simulink model "AXI_QPSK_Tx"  (R2017b)
settings: Solver=FixedStepAuto  StartTime=0.0  StopTime=1000/Rb  RelTol=1e-3
PreLoadFcn:
  | Rb = 10000;   % 1kbit / s
  | Rsym = Rb/2;   % 2 bits per symbol
  | Rsymbol = Rb/2;
  | OSR = 32;
  | f_error = 120;
  | 
  | design_filters_tx
values from neighbouring files (symbols this model uses):
  CIC_fine_Tx = 2^-(CIC_right_shift - CIC_left_shift - CIC_shift_Tx)    [design_filters_tx.m]
  fCIC = fCICcomp * R_CIC    (= 25600000)    [design_filters_tx.m]
  fHB = fRRC * R_HB    (= 40000)    [design_filters_tx.m]
  R_CIC = 320    [design_filters_tx.m]
  R_CICcomp = 2    [design_filters_tx.m]
  R_HB = 2    [design_filters_tx.m]
  R_RRC = 4    [design_filters_tx.m]
undefined symbols (not defined in the file or in its folder): AXI4, Lite
libraries: xbsIndex_r4 x281, hdlsllib x2
(part 2 of 3)

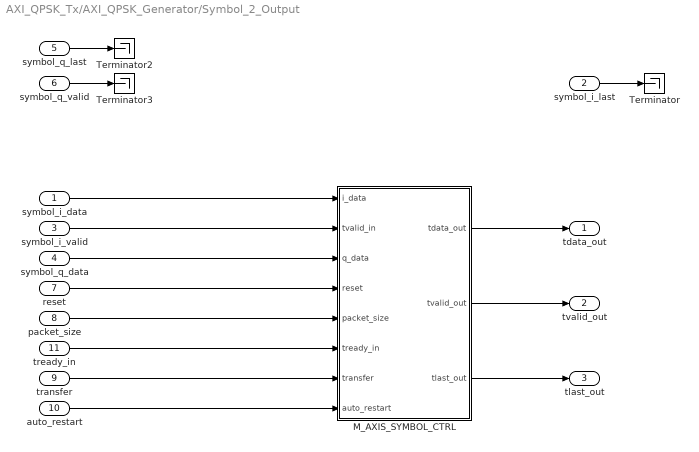
== system AXI_QPSK_Tx/AXI_QPSK_Generator/Symbol_2_Output ==
  symbol_i_data : Inport
  symbol_i_last : Inport  Port=2
  symbol_i_valid : Inport  Port=3
  symbol_q_data : Inport  Port=4
  symbol_q_last : Inport  Port=5
  symbol_q_valid : Inport  Port=6
  reset : Inport  Port=7
  packet_size : Inport  Port=8
  transfer : Inport  Port=9
  auto_restart : Inport  Port=10
  tready_in : Inport  Port=11
  M_AXIS_SYMBOL_CTRL : Subsystem
  Terminator : Terminator
  Terminator2 : Terminator
  Terminator3 : Terminator
  tdata_out : Outport
  tvalid_out : Outport  Port=2
  tlast_out : Outport  Port=3
  wires:
  symbol_i_last/1 -> Terminator/1
  symbol_q_last/1 -> Terminator2/1
  symbol_q_valid/1 -> Terminator3/1
  symbol_i_data/1 -> M_AXIS_SYMBOL_CTRL/1(i_data)
  symbol_i_valid/1 -> M_AXIS_SYMBOL_CTRL/2(tvalid_in)
  symbol_q_data/1 -> M_AXIS_SYMBOL_CTRL/3(q_data)
  reset/1 -> M_AXIS_SYMBOL_CTRL/4(reset)
  packet_size/1 -> M_AXIS_SYMBOL_CTRL/5(packet_size)
  tready_in/1 -> M_AXIS_SYMBOL_CTRL/6(tready_in)
  M_AXIS_SYMBOL_CTRL/1(tdata_out) -> tdata_out/1
  M_AXIS_SYMBOL_CTRL/2(tvalid_out) -> tvalid_out/1
  M_AXIS_SYMBOL_CTRL/3(tlast_out) -> tlast_out/1
  transfer/1 -> M_AXIS_SYMBOL_CTRL/7(transfer)
  auto_restart/1 -> M_AXIS_SYMBOL_CTRL/8(auto_restart)

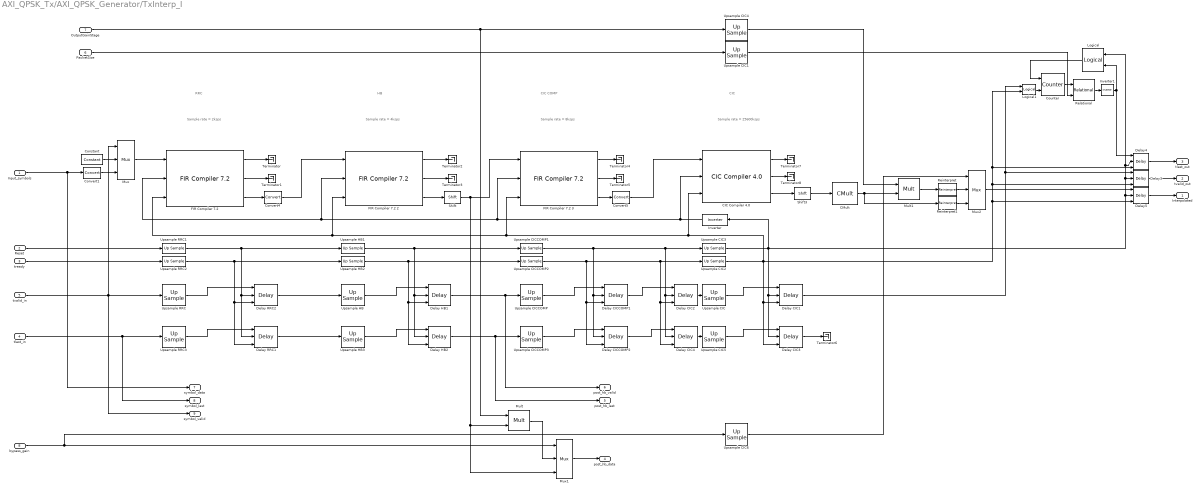
== system AXI_QPSK_Tx/AXI_QPSK_Generator/TxInterp_I ==
  note: HB
  note: RRC
  note: CIC COMP
  note: CIC
  note: Sample rate
      | = 2ksps
  note: Sample rate
      | = 4ksps
  note: Sample rate
      | = 8ksps
  note: Sample rate
      | = 25600ksps
  Input_symbols : Inport
  Reset : Inport  Port=2
  tready : Inport  Port=3
  tlast_in : Inport  Port=4
  tvalid_in : Inport  Port=5
  PacketSize : Inport  Port=6
  OutputGainStage : Inport  Port=7
  bypass_gain : Inport  Port=8
  "CIC Compiler 4.0 " : xbsIndex_r4/CIC Compiler 4.0   filter_type=Interpolation  number_of_stages=5  differential_delay=1  number_of_channels=1  sample_rate_changes=Fixed  fixed_or_initial_rate=R_CIC  minimum_rate=3200  maximum_rate=3200  ratespecification=Maximum_Possible  sampleperiod=3200  hardwareoversamplingrate=1  quantization=Full_Precision  output_data_width=65  use_xtreme_dsp_slice=on  use_streaming_interface=on  has_aclken=on  has_aresetn=on  has_dout_tready=off  trim_axipin_name=on  gui_behaviour=Sysgen_GUI  input_data_width=18  ip_name=CIC Compiler  ip_version=4.0  dsptool_ready=true  wrapper_available=true  port_translation_map={ 'aclken' => 'en', 'aresetn' => 'rst' }  ipcore_xco_need_fpga_part=true  ipcore_verbose=false  block_type=cic_compiler_v4_0
  CMult : xbsIndex_r4/CMult  const=CIC_fine_Tx  gui_display_data_type=Fixed-point  const_n_bits=16  const_bin_pt=15  float_type=Single  exp_bits=8  fraction_bits=24  en=off  latency=0  precision=User Defined  arith_type="Signed  (2's comp)"  n_bits=16  bin_pt=15  quantization=Truncate  overflow=Wrap  use_behavioral_HDL=off  mem_type=Distributed RAM  pipeline=off  dbl_ovrd=off  block_type=cmult
  Constant : xbsIndex_r4/Constant  const=0  gui_display_data_type=Fixed-point  arith_type=Signed (2's comp)  n_bits=16  bin_pt=0  preci_type=Single  exp_width=8  frac_width=24  explicit_period=on  period=2/Rb  equ=P=C  opselect=C  inp2=PCIN>>17  opr=+  inp1=P  carry=CIN  dbl_ovrd=off  block_type=constant
  Convert1 : xbsIndex_r4/Convert  gui_display_data_type=Fixed-point  arith_type="Signed  (2's comp)"  n_bits=16  bin_pt=0  float_type=Single  exp_bits=8  fraction_bits=24  quantization=Truncate  overflow=Wrap  en=off  latency=0  pipeline=off  dbl_ovrd=off  block_type=convert
  Convert4 : xbsIndex_r4/Convert  gui_display_data_type=Fixed-point  arith_type="Signed  (2's comp)"  n_bits=16  bin_pt=15  float_type=Single  exp_bits=8  fraction_bits=24  quantization=Truncate  overflow=Wrap  en=off  latency=0  pipeline=off  dbl_ovrd=off  block_type=convert
  Convert5 : xbsIndex_r4/Convert  gui_display_data_type=Fixed-point  arith_type="Signed  (2's comp)"  n_bits=16  bin_pt=15  float_type=Single  exp_bits=8  fraction_bits=24  quantization=Truncate  overflow=Wrap  en=off  latency=0  pipeline=off  dbl_ovrd=off  block_type=convert
  Counter : xbsIndex_r4/Counter  cnt_type=Free Running  cnt_to=Inf  operation=Up  start_count=0  cnt_by_val=1  arith_type=Unsigned  n_bits=32  bin_pt=0  load_pin=off  rst=on  en=on  explicit_period=on  period=1/fCIC  use_behavioral_HDL=off  implementation=Fabric  dbl_ovrd=off  block_type=counter
  Delay CIC1 : xbsIndex_r4/Delay  rst=on  infoeditControl=Selection of Reset will increase slice count due to use of real FFs and instead of SRLs  en=on  latency=3*8  reg_retiming=off  dbl_ovrd=off  block_type=delay
  Delay CIC2 : xbsIndex_r4/Delay  rst=on  infoeditControl=Selection of Reset will increase slice count due to use of real FFs and instead of SRLs  en=on  latency=4  reg_retiming=off  dbl_ovrd=off  block_type=delay
  Delay CIC3 : xbsIndex_r4/Delay  rst=on  infoeditControl=Selection of Reset will increase slice count due to use of real FFs and instead of SRLs  en=on  latency=3*8-1  reg_retiming=off  dbl_ovrd=off  block_type=delay
  Delay CIC4 : xbsIndex_r4/Delay  rst=on  infoeditControl=Selection of Reset will increase slice count due to use of real FFs and instead of SRLs  en=on  latency=5  reg_retiming=off  dbl_ovrd=off  block_type=delay
  Delay CICCOMP1 : xbsIndex_r4/Delay  rst=on  infoeditControl=Selection of Reset will increase slice count due to use of real FFs and instead of SRLs  en=on  latency=R_CICcomp*4  reg_retiming=off  dbl_ovrd=off  block_type=delay
  Delay CICCOMP2 : xbsIndex_r4/Delay  rst=on  infoeditControl=Selection of Reset will increase slice count due to use of real FFs and instead of SRLs  en=on  latency=R_CICcomp*4+1  reg_retiming=off  dbl_ovrd=off  block_type=delay
  Delay HB1 : xbsIndex_r4/Delay  rst=on  infoeditControl=Selection of Reset will increase slice count due to use of real FFs and instead of SRLs  en=on  latency=R_HB*2  reg_retiming=off  dbl_ovrd=off  block_type=delay
  Delay HB2 : xbsIndex_r4/Delay  rst=on  infoeditControl=Selection of Reset will increase slice count due to use of real FFs and instead of SRLs  en=on  latency=R_HB*2+1  reg_retiming=off  dbl_ovrd=off  block_type=delay
  Delay RRC1 : xbsIndex_r4/Delay  rst=on  infoeditControl=Selection of Reset will increase slice count due to use of real FFs and instead of SRLs  en=on  latency=3*R_RRC  reg_retiming=off  dbl_ovrd=off  block_type=delay
  Delay RRC2 : xbsIndex_r4/Delay  rst=on  infoeditControl=Selection of Reset will increase slice count due to use of real FFs and instead of SRLs  en=on  latency=R_RRC*2+1  reg_retiming=off  dbl_ovrd=off  block_type=delay
  Delay3 : xbsIndex_r4/Delay  rst=on  infoeditControl=Selection of Reset will increase slice count due to use of real FFs and instead of SRLs  en=on  latency=1  reg_retiming=off  dbl_ovrd=off  block_type=delay
  Delay4 : xbsIndex_r4/Delay  rst=on  infoeditControl=Selection of Reset will increase slice count due to use of real FFs and instead of SRLs  en=on  latency=1  reg_retiming=off  dbl_ovrd=off  block_type=delay
  Delay5 : xbsIndex_r4/Delay  rst=on  infoeditControl=Selection of Reset will increase slice count due to use of real FFs and instead of SRLs  en=on  latency=1  reg_retiming=off  dbl_ovrd=off  block_type=delay
  "FIR Compiler 7.2 " : xbsIndex_r4/FIR Compiler 7.2   coefficientvector=WRRC.Numerator  coefficient_sets=1  coefficient_reload=off  filter_type=Interpolation  rate_change_type=Integer  interpolation_rate=R_RRC  decimation_rate=1  zero_pack_factor=1  channel_sequence=Basic  number_channels=1  pattern_list='P4-0,P4-1,P4-2,P4-3,P4-4'  number_paths=1  ratespecification=Maximum_Possible  sampleperiod=1  hardwareoversamplingrate=1  coefficient_sign=Signed  quantization=Quantize_Only  coefficient_width=16  bestprecision=on  coefficient_fractional_bits=15  coefficient_structure=Inferred  output_rounding_mode=Full_Precision  output_width=31  filter_architecture=Systolic_Multiply_Accumulate  optimization_goal=Area  optimization_list='None'  data_buffer_type=Automatic  coefficient_buffer_type=Automatic  input_buffer_type=Automatic  output_buffer_type=Automatic  preference_for_other_storage=Automatic  multi_column_support=Automatic  columnconfig='13'  inter_column_pipe_length=4  data_has_tlast=Not_Required  m_data_has_tready=off  s_data_has_fifo=off  s_data_has_tuser=Not_Required  m_data_has_tuser=Not_Required  s_config_sync_mode=On_Vector  s_config_method=Single  num_reload_slots=1  has_aclken=on  has_aresetn=on  infoeditControl=ARESETn must be asserted for a minimum of 2 cycles  reset_data_vector=on  trim_axipin_name=on  simulation_type=hybrid_sim  simulation_model=sysgen:xfirv7_2_cmodel  data_path_portlist={ 's_axis_data_tdata', 'm_axis_data_tdata' }  passband_min=0.0  passband_max=0.5  stopband_min=0.5  stopband_max=1.0  filter_selection=1  gui_behaviour='Sysgen_GUI'  data_sign=Signed  data_width=16  data_fractional_bits=0  data_tuser_width=1  wrapper_available=true  ip_wrap_arbitrary_binary_point=true  ip_name=FIR Compiler  ip_version=7.2  dsptool_ready=true  ipcore_usecache=true  ipcore_useipmodelcache=true  port_translation_map={ 'aclken' => 'en', 'aresetn' => 'rst' }  run_core_at_system_period=true  ipcore_xco_need_fpga_part=true  block_type=fir_compiler_v7_2
      settings: infoedit=Maximum Possible : Maximizes oversampling rate. Abstracted input handshake (no s_data_tvalid) and automatic rate propagation.<br>Hardware Oversampling Rate : Specifies oversampling rate relative to the input sample period. Abstracted input handshake (no s_data_tvalid) and automatic rate propagation.<br>Input/Output Sample Period : Specifies absolute oversampling rate. No input handshake abstraction (exposes s_data_tvalid) and no rate propagation.
  FIR Compiler 7.2 2 : xbsIndex_r4/FIR Compiler 7.2   coefficientvector=HB.Numerator  coefficient_sets=1  coefficient_reload=off  filter_type=Interpolation  rate_change_type=Integer  interpolation_rate=2  decimation_rate=1  zero_pack_factor=1  channel_sequence=Basic  number_channels=1  pattern_list='P4-0,P4-1,P4-2,P4-3,P4-4'  number_paths=1  ratespecification=Maximum_Possible  sampleperiod=1  hardwareoversamplingrate=1  coefficient_sign=Signed  quantization=Quantize_Only  coefficient_width=16  bestprecision=on  coefficient_fractional_bits=15  coefficient_structure=Inferred  output_rounding_mode=Full_Precision  output_width=32  filter_architecture=Systolic_Multiply_Accumulate  optimization_goal=Area  optimization_list='None'  data_buffer_type=Automatic  coefficient_buffer_type=Automatic  input_buffer_type=Automatic  output_buffer_type=Automatic  preference_for_other_storage=Automatic  multi_column_support=Automatic  columnconfig='6'  inter_column_pipe_length=4  data_has_tlast=Not_Required  m_data_has_tready=off  s_data_has_fifo=off  s_data_has_tuser=Not_Required  m_data_has_tuser=Not_Required  s_config_sync_mode=On_Vector  s_config_method=Single  num_reload_slots=1  has_aclken=on  has_aresetn=on  infoeditControl=ARESETn must be asserted for a minimum of 2 cycles  reset_data_vector=on  trim_axipin_name=on  simulation_type=hybrid_sim  simulation_model=sysgen:xfirv7_2_cmodel  data_path_portlist={ 's_axis_data_tdata', 'm_axis_data_tdata' }  passband_min=0.0  passband_max=0.5  stopband_min=0.5  stopband_max=1.0  filter_selection=1  gui_behaviour='Sysgen_GUI'  data_sign=Signed  data_width=16  data_fractional_bits=0  data_tuser_width=1  wrapper_available=true  ip_wrap_arbitrary_binary_point=true  ip_name=FIR Compiler  ip_version=7.2  dsptool_ready=true  ipcore_usecache=true  ipcore_useipmodelcache=true  port_translation_map={ 'aclken' => 'en', 'aresetn' => 'rst' }  run_core_at_system_period=true  ipcore_xco_need_fpga_part=true  block_type=fir_compiler_v7_2
      settings: infoedit=Maximum Possible : Maximizes oversampling rate. Abstracted input handshake (no s_data_tvalid) and automatic rate propagation.<br>Hardware Oversampling Rate : Specifies oversampling rate relative to the input sample period. Abstracted input handshake (no s_data_tvalid) and automatic rate propagation.<br>Input/Output Sample Period : Specifies absolute oversampling rate. No input handshake abstraction (exposes s_data_tvalid) and no rate propagation.
  FIR Compiler 7.2 3 : xbsIndex_r4/FIR Compiler 7.2   coefficientvector=WComp.Numerator  coefficient_sets=1  coefficient_reload=off  filter_type=Interpolation  rate_change_type=Integer  interpolation_rate=R_CICcomp  decimation_rate=1  zero_pack_factor=1  channel_sequence=Basic  number_channels=1  pattern_list='P4-0,P4-1,P4-2,P4-3,P4-4'  number_paths=1  ratespecification=Maximum_Possible  sampleperiod=1  hardwareoversamplingrate=1  coefficient_sign=Signed  quantization=Quantize_Only  coefficient_width=16  bestprecision=on  coefficient_fractional_bits=15  coefficient_structure=Inferred  output_rounding_mode=Full_Precision  output_width=33  filter_architecture=Systolic_Multiply_Accumulate  optimization_goal=Area  optimization_list='None'  data_buffer_type=Automatic  coefficient_buffer_type=Automatic  input_buffer_type=Automatic  output_buffer_type=Automatic  preference_for_other_storage=Automatic  multi_column_support=Automatic  columnconfig='19'  inter_column_pipe_length=4  data_has_tlast=Not_Required  m_data_has_tready=off  s_data_has_fifo=off  s_data_has_tuser=Not_Required  m_data_has_tuser=Not_Required  s_config_sync_mode=On_Vector  s_config_method=Single  num_reload_slots=1  has_aclken=on  has_aresetn=on  infoeditControl=ARESETn must be asserted for a minimum of 2 cycles  reset_data_vector=on  trim_axipin_name=on  simulation_type=hybrid_sim  simulation_model=sysgen:xfirv7_2_cmodel  data_path_portlist={ 's_axis_data_tdata', 'm_axis_data_tdata' }  passband_min=0.0  passband_max=0.5  stopband_min=0.5  stopband_max=1.0  filter_selection=1  gui_behaviour='Sysgen_GUI'  data_sign=Signed  data_width=16  data_fractional_bits=0  data_tuser_width=1  wrapper_available=true  ip_wrap_arbitrary_binary_point=true  ip_name=FIR Compiler  ip_version=7.2  dsptool_ready=true  ipcore_usecache=true  ipcore_useipmodelcache=true  port_translation_map={ 'aclken' => 'en', 'aresetn' => 'rst' }  run_core_at_system_period=true  ipcore_xco_need_fpga_part=true  block_type=fir_compiler_v7_2
      settings: infoedit=Maximum Possible : Maximizes oversampling rate. Abstracted input handshake (no s_data_tvalid) and automatic rate propagation.<br>Hardware Oversampling Rate : Specifies oversampling rate relative to the input sample period. Abstracted input handshake (no s_data_tvalid) and automatic rate propagation.<br>Input/Output Sample Period : Specifies absolute oversampling rate. No input handshake abstraction (exposes s_data_tvalid) and no rate propagation.
  Inverter : xbsIndex_r4/Inverter  en=off  latency=0  dbl_ovrd=off  block_type=inv
  Inverter1 : xbsIndex_r4/Inverter  en=off  latency=0  dbl_ovrd=off  block_type=inv
  Logical : xbsIndex_r4/Logical  logical_function=OR  inputs=2  en=off  latency=0  precision=Full  arith_type=Unsigned  n_bits=16  bin_pt=0  align_bp=on  dbl_ovrd=off  block_type=logical
  Logical1 : xbsIndex_r4/Logical  logical_function=AND  inputs=2  en=off  latency=0  precision=Full  arith_type=Unsigned  n_bits=16  bin_pt=0  align_bp=on  dbl_ovrd=off  block_type=logical
  Mult : xbsIndex_r4/Mult  precision=User Defined  arith_type="Signed  (2's comp)"  n_bits=16  bin_pt=15  quantization=Truncate  overflow=Wrap  en=off  latency=0  use_behavioral_HDL=off  opt=Speed  use_embedded=on  optimum_pipeline=off  pipeline=on  dbl_ovrd=off  use_rpm=on  placement_style=Triangular  block_type=mult
  Mult1 : xbsIndex_r4/Mult  precision=User Defined  arith_type="Signed  (2's comp)"  n_bits=16  bin_pt=15  quantization=Truncate  overflow=Wrap  en=off  latency=0  use_behavioral_HDL=off  opt=Speed  use_embedded=on  optimum_pipeline=off  pipeline=on  dbl_ovrd=off  use_rpm=on  placement_style=Triangular  block_type=mult
  Mux : xbsIndex_r4/Mux  inputs=2  en=off  latency=0  precision=Full  arith_type=Unsigned  n_bits=16  bin_pt=14  quantization=Truncate  overflow=Wrap  dbl_ovrd=off  block_type=mux
  Mux1 : xbsIndex_r4/Mux  inputs=2  en=off  latency=0  precision=Full  arith_type=Unsigned  n_bits=16  bin_pt=14  quantization=Truncate  overflow=Wrap  dbl_ovrd=off  block_type=mux
  Mux2 : xbsIndex_r4/Mux  inputs=2  en=off  latency=0  precision=Full  arith_type=Unsigned  n_bits=16  bin_pt=14  quantization=Truncate  overflow=Wrap  dbl_ovrd=off  block_type=mux
  Reinterpret : xbsIndex_r4/Reinterpret  force_arith_type=on  arith_type=Unsigned  force_bin_pt=on  bin_pt=0  block_type=reinterpret
  Reinterpret1 : xbsIndex_r4/Reinterpret  force_arith_type=on  arith_type=Unsigned  force_bin_pt=on  bin_pt=0  block_type=reinterpret
  Relational : xbsIndex_r4/Relational  mode=a<b  op_type=Bool  en=off  latency=0  dbl_ovrd=off  block_type=relational
  Shift : xbsIndex_r4/Shift  shift_dir=Left  shift_bits=1  en=off  latency=0  precision=User Defined  arith_type="Signed  (2's comp)"  n_bits=16  bin_pt=15  quantization=Truncate  overflow=Wrap  dbl_ovrd=off  block_type=shift
  Shift3 : xbsIndex_r4/Shift  shift_dir=Right  shift_bits=CIC_shift_Tx  en=off  latency=0  precision=User Defined  arith_type="Signed  (2's comp)"  n_bits=17  bin_pt=14  quantization=Truncate  overflow=Wrap  dbl_ovrd=off  block_type=shift
  Terminator{,1..8} (9 alike) : Terminator
  Upsample CIC : xbsIndex_r4/Up Sample  sample_ratio=R_CIC  copy_samples=on  en=off  latency=0  dbl_ovrd=off  block_type=usamp
  Upsample CIC1 : xbsIndex_r4/Up Sample  sample_ratio=fCIC/(Rb/2)  copy_samples=on  en=off  latency=0  dbl_ovrd=off  block_type=usamp
  Upsample CIC2 : xbsIndex_r4/Up Sample  sample_ratio=R_CIC  copy_samples=on  en=off  latency=0  dbl_ovrd=off  block_type=usamp
  Upsample CIC3 : xbsIndex_r4/Up Sample  sample_ratio=R_CIC  copy_samples=on  en=off  latency=0  dbl_ovrd=off  block_type=usamp
  Upsample CIC4 : xbsIndex_r4/Up Sample  sample_ratio=fCIC/fHB  copy_samples=on  en=off  latency=0  dbl_ovrd=off  block_type=usamp
  Upsample CIC5 : xbsIndex_r4/Up Sample  sample_ratio=R_CIC  copy_samples=off  en=off  latency=0  dbl_ovrd=off  block_type=usamp
  Upsample CIC6 : xbsIndex_r4/Up Sample  sample_ratio=fCIC/fHB  copy_samples=on  en=off  latency=0  dbl_ovrd=off  block_type=usamp
  Upsample CICCOMP : xbsIndex_r4/Up Sample  sample_ratio=R_CICcomp  copy_samples=on  en=off  latency=0  dbl_ovrd=off  block_type=usamp
  Upsample CICCOMP1 : xbsIndex_r4/Up Sample  sample_ratio=R_CICcomp  copy_samples=on  en=off  latency=0  dbl_ovrd=off  block_type=usamp
  Upsample CICCOMP2 : xbsIndex_r4/Up Sample  sample_ratio=R_CICcomp  copy_samples=on  en=off  latency=0  dbl_ovrd=off  block_type=usamp
  Upsample CICCOMP3 : xbsIndex_r4/Up Sample  sample_ratio=R_CICcomp  copy_samples=off  en=off  latency=0  dbl_ovrd=off  block_type=usamp
  Upsample HB : xbsIndex_r4/Up Sample  sample_ratio=R_HB  copy_samples=on  en=off  latency=0  dbl_ovrd=off  block_type=usamp
  Upsample HB1 : xbsIndex_r4/Up Sample  sample_ratio=R_HB  copy_samples=on  en=off  latency=0  dbl_ovrd=off  block_type=usamp
  Upsample HB2 : xbsIndex_r4/Up Sample  sample_ratio=R_HB  copy_samples=on  en=off  latency=0  dbl_ovrd=off  block_type=usamp
  Upsample HB3 : xbsIndex_r4/Up Sample  sample_ratio=R_HB  copy_samples=off  en=off  latency=0  dbl_ovrd=off  block_type=usamp
  Upsample RRC : xbsIndex_r4/Up Sample  sample_ratio=R_RRC  copy_samples=on  en=off  latency=0  dbl_ovrd=off  block_type=usamp
  Upsample RRC1 : xbsIndex_r4/Up Sample  sample_ratio=R_RRC  copy_samples=on  en=off  latency=0  dbl_ovrd=off  block_type=usamp
  Upsample RRC2 : xbsIndex_r4/Up Sample  sample_ratio=R_RRC  copy_samples=on  en=off  latency=0  dbl_ovrd=off  block_type=usamp
  Upsample RRC3 : xbsIndex_r4/Up Sample  sample_ratio=R_RRC  copy_samples=off  en=off  latency=0  dbl_ovrd=off  block_type=usamp
  Interpolated : Outport
  tvalid_out : Outport  Port=2
  tlast_out : Outport  Port=3
  post_hb_data : Outport  Port=4
  post_hb_last : Outport  Port=5
  post_hb_valid : Outport  Port=6
  symbol_data : Outport  Port=7
  symbol_last : Outport  Port=8
  symbol_valid : Outport  Port=9
  wires:
  bypass_gain/1 -> Mux1/1, Upsample CIC6/1
  Reinterpret1/1 -> Mux2/3
  Mux2/1 -> Delay5/1
  Reinterpret/1 -> Mux2/2
  OutputGainStage/1 -> Mult/1, Upsample CIC4/1
  CMult/1 -> Reinterpret1/1, Mult1/2
  Shift/1 -> Mux1/3, Mult/2, FIR Compiler 7.2 3/1
  Convert1/1 -> Mux/3
  Convert4/1 -> FIR Compiler 7.2 2/1
  "CIC Compiler 4.0 "/3 -> Shift3/1
  Logical1/1 -> Counter/2
  Delay5/1 -> Interpolated/1
  Delay3/1 -> tvalid_out/1
  Delay4/1 -> tlast_out/1
  Relational/1 -> Inverter1/1
  Inverter1/1 -> Logical/2, Delay4/1
  Logical/1 -> Counter/1
  Counter/1 -> Relational/1
  Upsample CIC1/1 -> Relational/2
  PacketSize/1 -> Upsample CIC1/1
  "FIR Compiler 7.2 "/1 -> Terminator/1
  "FIR Compiler 7.2 "/2 -> Terminator1/1
  Shift3/1 -> CMult/1
  "FIR Compiler 7.2 "/3 -> Convert4/1
  FIR Compiler 7.2 2/3 -> Shift/1
  FIR Compiler 7.2 2/2 -> Terminator3/1
  FIR Compiler 7.2 2/1 -> Terminator2/1
  FIR Compiler 7.2 3/3 -> Convert5/1
  FIR Compiler 7.2 3/1 -> Terminator4/1
  FIR Compiler 7.2 3/2 -> Terminator5/1
  "CIC Compiler 4.0 "/1 -> Terminator7/1
  Convert5/1 -> "CIC Compiler 4.0 "/1
  Reset/1 -> Upsample RRC1/1
  Upsample CIC/1 -> Delay CIC1/1
  "CIC Compiler 4.0 "/2 -> Terminator8/1
  Upsample CIC2/1 -> Delay CIC3/3, Delay CIC1/3, Logical1/2, Delay4/3, Delay3/3, Delay5/3, "FIR Compiler 7.2 "/3, FIR Compiler 7.2 2/3, FIR Compiler 7.2 3/3, "CIC Compiler 4.0 "/3
  Upsample CIC3/1 -> Delay CIC3/2, Delay CIC1/2, Delay5/2, Delay3/2, Logical/1, Delay4/2, Inverter/1
  tvalid_in/1 -> Upsample RRC/1, symbol_valid/1, Mux/1
  Delay RRC2/1 -> Upsample HB/1
  Upsample RRC/1 -> Delay RRC2/1
  Upsample HB/1 -> Delay HB1/1
  Upsample CICCOMP/1 -> Delay CICCOMP1/1
  Delay CIC1/1 -> Logical1/1, Delay3/1
  tready/1 -> Upsample RRC2/1
  Upsample CICCOMP3/1 -> Delay CICCOMP2/1
  Upsample HB3/1 -> Delay HB2/1
  Upsample RRC3/1 -> Delay RRC1/1
  Delay RRC1/1 -> Upsample HB3/1
  tlast_in/1 -> Upsample RRC3/1, symbol_last/1
  Upsample CICCOMP2/1 -> Delay CICCOMP2/3, Delay CICCOMP1/3, Delay CIC4/3, Delay CIC2/3, Upsample CIC2/1
  Upsample CICCOMP1/1 -> Delay CICCOMP2/2, Delay CICCOMP1/2, Delay CIC4/2, Delay CIC2/2, Upsample CIC3/1
  Upsample HB2/1 -> Delay HB2/3, Delay HB1/3, Upsample CICCOMP2/1
  Upsample HB1/1 -> Delay HB2/2, Delay HB1/2, Upsample CICCOMP1/1
  Upsample RRC2/1 -> Delay RRC1/3, Delay RRC2/3, Upsample HB2/1
  Upsample RRC1/1 -> Delay RRC1/2, Delay RRC2/2, Upsample HB1/1
  Upsample CIC5/1 -> Delay CIC3/1
  Inverter/1 -> FIR Compiler 7.2 3/2, "FIR Compiler 7.2 "/2, FIR Compiler 7.2 2/2, "CIC Compiler 4.0 "/2
  Delay CIC2/1 -> Upsample CIC/1
  Delay CICCOMP1/1 -> Delay CIC2/1
  Delay CIC4/1 -> Upsample CIC5/1
  Delay CICCOMP2/1 -> Delay CIC4/1
  Mux/1 -> "FIR Compiler 7.2 "/1
  Input_symbols/1 -> Convert1/1, symbol_data/1
  Constant/1 -> Mux/2
  Delay HB2/1 -> Upsample CICCOMP3/1, post_hb_last/1
  Delay HB1/1 -> post_hb_valid/1, Upsample CICCOMP/1
  Delay CIC3/1 -> Terminator6/1
  Mult1/1 -> Reinterpret/1
  Upsample CIC4/1 -> Mult1/1
  Mux1/1 -> post_hb_data/1
  Mult/1 -> Mux1/2
  Upsample CIC6/1 -> Mux2/1

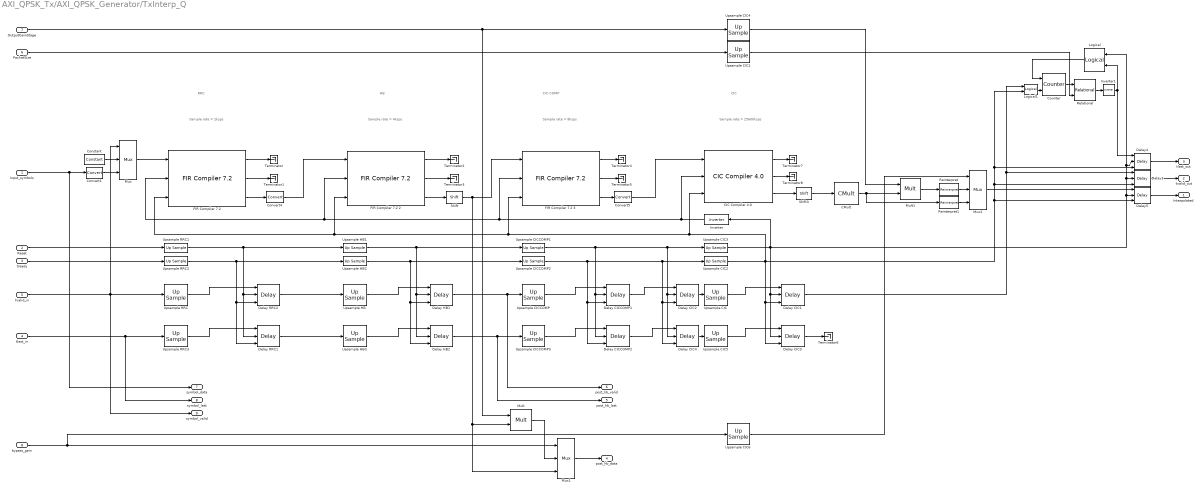
== system AXI_QPSK_Tx/AXI_QPSK_Generator/TxInterp_Q ==
  note: Sample rate
      | = 25600ksps
  note: Sample rate
      | = 8ksps
  note: Sample rate
      | = 4ksps
  note: Sample rate
      | = 2ksps
  note: CIC
  note: CIC COMP
  note: RRC
  note: HB
  Input_symbols : Inport
  Reset : Inport  Port=2
  tready : Inport  Port=3
  tlast_in : Inport  Port=4
  tvalid_in : Inport  Port=5
  PacketSize : Inport  Port=6
  OutputGainStage : Inport  Port=7
  bypass_gain : Inport  Port=8
  "CIC Compiler 4.0 " : xbsIndex_r4/CIC Compiler 4.0   filter_type=Interpolation  number_of_stages=5  differential_delay=1  number_of_channels=1  sample_rate_changes=Fixed  fixed_or_initial_rate=R_CIC  minimum_rate=3200  maximum_rate=3200  ratespecification=Maximum_Possible  sampleperiod=3200  hardwareoversamplingrate=1  quantization=Full_Precision  output_data_width=65  use_xtreme_dsp_slice=on  use_streaming_interface=on  has_aclken=on  has_aresetn=on  has_dout_tready=off  trim_axipin_name=on  gui_behaviour=Sysgen_GUI  input_data_width=18  ip_name=CIC Compiler  ip_version=4.0  dsptool_ready=true  wrapper_available=true  port_translation_map={ 'aclken' => 'en', 'aresetn' => 'rst' }  ipcore_xco_need_fpga_part=true  ipcore_verbose=false  block_type=cic_compiler_v4_0
  CMult : xbsIndex_r4/CMult  const=CIC_fine_Tx  gui_display_data_type=Fixed-point  const_n_bits=16  const_bin_pt=15  float_type=Single  exp_bits=8  fraction_bits=24  en=off  latency=0  precision=User Defined  arith_type="Signed  (2's comp)"  n_bits=16  bin_pt=15  quantization=Truncate  overflow=Wrap  use_behavioral_HDL=off  mem_type=Distributed RAM  pipeline=off  dbl_ovrd=off  block_type=cmult
  Constant : xbsIndex_r4/Constant  const=0  gui_display_data_type=Fixed-point  arith_type=Signed (2's comp)  n_bits=16  bin_pt=0  preci_type=Single  exp_width=8  frac_width=24  explicit_period=on  period=2/Rb  equ=P=C  opselect=C  inp2=PCIN>>17  opr=+  inp1=P  carry=CIN  dbl_ovrd=off  block_type=constant
  Convert1 : xbsIndex_r4/Convert  gui_display_data_type=Fixed-point  arith_type="Signed  (2's comp)"  n_bits=16  bin_pt=0  float_type=Single  exp_bits=8  fraction_bits=24  quantization=Truncate  overflow=Wrap  en=off  latency=0  pipeline=off  dbl_ovrd=off  block_type=convert
  Convert4 : xbsIndex_r4/Convert  gui_display_data_type=Fixed-point  arith_type="Signed  (2's comp)"  n_bits=16  bin_pt=15  float_type=Single  exp_bits=8  fraction_bits=24  quantization=Truncate  overflow=Wrap  en=off  latency=0  pipeline=off  dbl_ovrd=off  block_type=convert
  Convert5 : xbsIndex_r4/Convert  gui_display_data_type=Fixed-point  arith_type="Signed  (2's comp)"  n_bits=16  bin_pt=15  float_type=Single  exp_bits=8  fraction_bits=24  quantization=Truncate  overflow=Wrap  en=off  latency=0  pipeline=off  dbl_ovrd=off  block_type=convert
  Counter : xbsIndex_r4/Counter  cnt_type=Free Running  cnt_to=Inf  operation=Up  start_count=0  cnt_by_val=1  arith_type=Unsigned  n_bits=32  bin_pt=0  load_pin=off  rst=on  en=on  explicit_period=on  period=1/fCIC  use_behavioral_HDL=off  implementation=Fabric  dbl_ovrd=off  block_type=counter
  Delay CIC1 : xbsIndex_r4/Delay  rst=on  infoeditControl=Selection of Reset will increase slice count due to use of real FFs and instead of SRLs  en=on  latency=3*8  reg_retiming=off  dbl_ovrd=off  block_type=delay
  Delay CIC2 : xbsIndex_r4/Delay  rst=on  infoeditControl=Selection of Reset will increase slice count due to use of real FFs and instead of SRLs  en=on  latency=4  reg_retiming=off  dbl_ovrd=off  block_type=delay
  Delay CIC3 : xbsIndex_r4/Delay  rst=on  infoeditControl=Selection of Reset will increase slice count due to use of real FFs and instead of SRLs  en=on  latency=3*8-1  reg_retiming=off  dbl_ovrd=off  block_type=delay
  Delay CIC4 : xbsIndex_r4/Delay  rst=on  infoeditControl=Selection of Reset will increase slice count due to use of real FFs and instead of SRLs  en=on  latency=5  reg_retiming=off  dbl_ovrd=off  block_type=delay
  Delay CICCOMP1 : xbsIndex_r4/Delay  rst=on  infoeditControl=Selection of Reset will increase slice count due to use of real FFs and instead of SRLs  en=on  latency=R_CICcomp*4  reg_retiming=off  dbl_ovrd=off  block_type=delay
  Delay CICCOMP2 : xbsIndex_r4/Delay  rst=on  infoeditControl=Selection of Reset will increase slice count due to use of real FFs and instead of SRLs  en=on  latency=R_CICcomp*4+1  reg_retiming=off  dbl_ovrd=off  block_type=delay
  Delay HB1 : xbsIndex_r4/Delay  rst=on  infoeditControl=Selection of Reset will increase slice count due to use of real FFs and instead of SRLs  en=on  latency=R_HB*2  reg_retiming=off  dbl_ovrd=off  block_type=delay
  Delay HB2 : xbsIndex_r4/Delay  rst=on  infoeditControl=Selection of Reset will increase slice count due to use of real FFs and instead of SRLs  en=on  latency=R_HB*2+1  reg_retiming=off  dbl_ovrd=off  block_type=delay
  Delay RRC1 : xbsIndex_r4/Delay  rst=on  infoeditControl=Selection of Reset will increase slice count due to use of real FFs and instead of SRLs  en=on  latency=3*R_RRC  reg_retiming=off  dbl_ovrd=off  block_type=delay
  Delay RRC2 : xbsIndex_r4/Delay  rst=on  infoeditControl=Selection of Reset will increase slice count due to use of real FFs and instead of SRLs  en=on  latency=R_RRC*2+1  reg_retiming=off  dbl_ovrd=off  block_type=delay
  Delay3 : xbsIndex_r4/Delay  rst=on  infoeditControl=Selection of Reset will increase slice count due to use of real FFs and instead of SRLs  en=on  latency=1  reg_retiming=off  dbl_ovrd=off  block_type=delay
  Delay4 : xbsIndex_r4/Delay  rst=on  infoeditControl=Selection of Reset will increase slice count due to use of real FFs and instead of SRLs  en=on  latency=1  reg_retiming=off  dbl_ovrd=off  block_type=delay
  Delay5 : xbsIndex_r4/Delay  rst=on  infoeditControl=Selection of Reset will increase slice count due to use of real FFs and instead of SRLs  en=on  latency=1  reg_retiming=off  dbl_ovrd=off  block_type=delay
  "FIR Compiler 7.2 " : xbsIndex_r4/FIR Compiler 7.2   coefficientvector=WRRC.Numerator  coefficient_sets=1  coefficient_reload=off  filter_type=Interpolation  rate_change_type=Integer  interpolation_rate=R_RRC  decimation_rate=1  zero_pack_factor=1  channel_sequence=Basic  number_channels=1  pattern_list='P4-0,P4-1,P4-2,P4-3,P4-4'  number_paths=1  ratespecification=Maximum_Possible  sampleperiod=1  hardwareoversamplingrate=1  coefficient_sign=Signed  quantization=Quantize_Only  coefficient_width=16  bestprecision=on  coefficient_fractional_bits=15  coefficient_structure=Inferred  output_rounding_mode=Full_Precision  output_width=31  filter_architecture=Systolic_Multiply_Accumulate  optimization_goal=Area  optimization_list='None'  data_buffer_type=Automatic  coefficient_buffer_type=Automatic  input_buffer_type=Automatic  output_buffer_type=Automatic  preference_for_other_storage=Automatic  multi_column_support=Automatic  columnconfig='13'  inter_column_pipe_length=4  data_has_tlast=Not_Required  m_data_has_tready=off  s_data_has_fifo=off  s_data_has_tuser=Not_Required  m_data_has_tuser=Not_Required  s_config_sync_mode=On_Vector  s_config_method=Single  num_reload_slots=1  has_aclken=on  has_aresetn=on  infoeditControl=ARESETn must be asserted for a minimum of 2 cycles  reset_data_vector=on  trim_axipin_name=on  simulation_type=hybrid_sim  simulation_model=sysgen:xfirv7_2_cmodel  data_path_portlist={ 's_axis_data_tdata', 'm_axis_data_tdata' }  passband_min=0.0  passband_max=0.5  stopband_min=0.5  stopband_max=1.0  filter_selection=1  gui_behaviour='Sysgen_GUI'  data_sign=Signed  data_width=16  data_fractional_bits=0  data_tuser_width=1  wrapper_available=true  ip_wrap_arbitrary_binary_point=true  ip_name=FIR Compiler  ip_version=7.2  dsptool_ready=true  ipcore_usecache=true  ipcore_useipmodelcache=true  port_translation_map={ 'aclken' => 'en', 'aresetn' => 'rst' }  run_core_at_system_period=true  ipcore_xco_need_fpga_part=true  block_type=fir_compiler_v7_2
      settings: infoedit=Maximum Possible : Maximizes oversampling rate. Abstracted input handshake (no s_data_tvalid) and automatic rate propagation.<br>Hardware Oversampling Rate : Specifies oversampling rate relative to the input sample period. Abstracted input handshake (no s_data_tvalid) and automatic rate propagation.<br>Input/Output Sample Period : Specifies absolute oversampling rate. No input handshake abstraction (exposes s_data_tvalid) and no rate propagation.
  FIR Compiler 7.2 2 : xbsIndex_r4/FIR Compiler 7.2   coefficientvector=HB.Numerator  coefficient_sets=1  coefficient_reload=off  filter_type=Interpolation  rate_change_type=Integer  interpolation_rate=2  decimation_rate=1  zero_pack_factor=1  channel_sequence=Basic  number_channels=1  pattern_list='P4-0,P4-1,P4-2,P4-3,P4-4'  number_paths=1  ratespecification=Maximum_Possible  sampleperiod=1  hardwareoversamplingrate=1  coefficient_sign=Signed  quantization=Quantize_Only  coefficient_width=16  bestprecision=on  coefficient_fractional_bits=15  coefficient_structure=Inferred  output_rounding_mode=Full_Precision  output_width=32  filter_architecture=Systolic_Multiply_Accumulate  optimization_goal=Area  optimization_list='None'  data_buffer_type=Automatic  coefficient_buffer_type=Automatic  input_buffer_type=Automatic  output_buffer_type=Automatic  preference_for_other_storage=Automatic  multi_column_support=Automatic  columnconfig='6'  inter_column_pipe_length=4  data_has_tlast=Not_Required  m_data_has_tready=off  s_data_has_fifo=off  s_data_has_tuser=Not_Required  m_data_has_tuser=Not_Required  s_config_sync_mode=On_Vector  s_config_method=Single  num_reload_slots=1  has_aclken=on  has_aresetn=on  infoeditControl=ARESETn must be asserted for a minimum of 2 cycles  reset_data_vector=on  trim_axipin_name=on  simulation_type=hybrid_sim  simulation_model=sysgen:xfirv7_2_cmodel  data_path_portlist={ 's_axis_data_tdata', 'm_axis_data_tdata' }  passband_min=0.0  passband_max=0.5  stopband_min=0.5  stopband_max=1.0  filter_selection=1  gui_behaviour='Sysgen_GUI'  data_sign=Signed  data_width=16  data_fractional_bits=0  data_tuser_width=1  wrapper_available=true  ip_wrap_arbitrary_binary_point=true  ip_name=FIR Compiler  ip_version=7.2  dsptool_ready=true  ipcore_usecache=true  ipcore_useipmodelcache=true  port_translation_map={ 'aclken' => 'en', 'aresetn' => 'rst' }  run_core_at_system_period=true  ipcore_xco_need_fpga_part=true  block_type=fir_compiler_v7_2
      settings: infoedit=Maximum Possible : Maximizes oversampling rate. Abstracted input handshake (no s_data_tvalid) and automatic rate propagation.<br>Hardware Oversampling Rate : Specifies oversampling rate relative to the input sample period. Abstracted input handshake (no s_data_tvalid) and automatic rate propagation.<br>Input/Output Sample Period : Specifies absolute oversampling rate. No input handshake abstraction (exposes s_data_tvalid) and no rate propagation.
  FIR Compiler 7.2 3 : xbsIndex_r4/FIR Compiler 7.2   coefficientvector=WComp.Numerator  coefficient_sets=1  coefficient_reload=off  filter_type=Interpolation  rate_change_type=Integer  interpolation_rate=R_CICcomp  decimation_rate=1  zero_pack_factor=1  channel_sequence=Basic  number_channels=1  pattern_list='P4-0,P4-1,P4-2,P4-3,P4-4'  number_paths=1  ratespecification=Maximum_Possible  sampleperiod=1  hardwareoversamplingrate=1  coefficient_sign=Signed  quantization=Quantize_Only  coefficient_width=16  bestprecision=on  coefficient_fractional_bits=15  coefficient_structure=Inferred  output_rounding_mode=Full_Precision  output_width=33  filter_architecture=Systolic_Multiply_Accumulate  optimization_goal=Area  optimization_list='None'  data_buffer_type=Automatic  coefficient_buffer_type=Automatic  input_buffer_type=Automatic  output_buffer_type=Automatic  preference_for_other_storage=Automatic  multi_column_support=Automatic  columnconfig='19'  inter_column_pipe_length=4  data_has_tlast=Not_Required  m_data_has_tready=off  s_data_has_fifo=off  s_data_has_tuser=Not_Required  m_data_has_tuser=Not_Required  s_config_sync_mode=On_Vector  s_config_method=Single  num_reload_slots=1  has_aclken=on  has_aresetn=on  infoeditControl=ARESETn must be asserted for a minimum of 2 cycles  reset_data_vector=on  trim_axipin_name=on  simulation_type=hybrid_sim  simulation_model=sysgen:xfirv7_2_cmodel  data_path_portlist={ 's_axis_data_tdata', 'm_axis_data_tdata' }  passband_min=0.0  passband_max=0.5  stopband_min=0.5  stopband_max=1.0  filter_selection=1  gui_behaviour='Sysgen_GUI'  data_sign=Signed  data_width=16  data_fractional_bits=0  data_tuser_width=1  wrapper_available=true  ip_wrap_arbitrary_binary_point=true  ip_name=FIR Compiler  ip_version=7.2  dsptool_ready=true  ipcore_usecache=true  ipcore_useipmodelcache=true  port_translation_map={ 'aclken' => 'en', 'aresetn' => 'rst' }  run_core_at_system_period=true  ipcore_xco_need_fpga_part=true  block_type=fir_compiler_v7_2
      settings: infoedit=Maximum Possible : Maximizes oversampling rate. Abstracted input handshake (no s_data_tvalid) and automatic rate propagation.<br>Hardware Oversampling Rate : Specifies oversampling rate relative to the input sample period. Abstracted input handshake (no s_data_tvalid) and automatic rate propagation.<br>Input/Output Sample Period : Specifies absolute oversampling rate. No input handshake abstraction (exposes s_data_tvalid) and no rate propagation.
  Inverter : xbsIndex_r4/Inverter  en=off  latency=0  dbl_ovrd=off  block_type=inv
  Inverter1 : xbsIndex_r4/Inverter  en=off  latency=0  dbl_ovrd=off  block_type=inv
  Logical : xbsIndex_r4/Logical  logical_function=OR  inputs=2  en=off  latency=0  precision=Full  arith_type=Unsigned  n_bits=16  bin_pt=0  align_bp=on  dbl_ovrd=off  block_type=logical
  Logical1 : xbsIndex_r4/Logical  logical_function=AND  inputs=2  en=off  latency=0  precision=Full  arith_type=Unsigned  n_bits=16  bin_pt=0  align_bp=on  dbl_ovrd=off  block_type=logical
  Mult : xbsIndex_r4/Mult  precision=User Defined  arith_type="Signed  (2's comp)"  n_bits=16  bin_pt=15  quantization=Truncate  overflow=Wrap  en=off  latency=0  use_behavioral_HDL=off  opt=Speed  use_embedded=on  optimum_pipeline=off  pipeline=on  dbl_ovrd=off  use_rpm=on  placement_style=Triangular  block_type=mult
  Mult1 : xbsIndex_r4/Mult  precision=User Defined  arith_type="Signed  (2's comp)"  n_bits=16  bin_pt=15  quantization=Truncate  overflow=Wrap  en=off  latency=0  use_behavioral_HDL=off  opt=Speed  use_embedded=on  optimum_pipeline=off  pipeline=on  dbl_ovrd=off  use_rpm=on  placement_style=Triangular  block_type=mult
  Mux : xbsIndex_r4/Mux  inputs=2  en=off  latency=0  precision=Full  arith_type=Unsigned  n_bits=16  bin_pt=14  quantization=Truncate  overflow=Wrap  dbl_ovrd=off  block_type=mux
  Mux1 : xbsIndex_r4/Mux  inputs=2  en=off  latency=0  precision=Full  arith_type=Unsigned  n_bits=16  bin_pt=14  quantization=Truncate  overflow=Wrap  dbl_ovrd=off  block_type=mux
  Mux2 : xbsIndex_r4/Mux  inputs=2  en=off  latency=0  precision=Full  arith_type=Unsigned  n_bits=16  bin_pt=14  quantization=Truncate  overflow=Wrap  dbl_ovrd=off  block_type=mux
  Reinterpret : xbsIndex_r4/Reinterpret  force_arith_type=on  arith_type=Unsigned  force_bin_pt=on  bin_pt=0  block_type=reinterpret
  Reinterpret1 : xbsIndex_r4/Reinterpret  force_arith_type=on  arith_type=Unsigned  force_bin_pt=on  bin_pt=0  block_type=reinterpret
  Relational : xbsIndex_r4/Relational  mode=a<b  op_type=Bool  en=off  latency=0  dbl_ovrd=off  block_type=relational
  Shift : xbsIndex_r4/Shift  shift_dir=Left  shift_bits=1  en=off  latency=0  precision=User Defined  arith_type="Signed  (2's comp)"  n_bits=16  bin_pt=15  quantization=Truncate  overflow=Wrap  dbl_ovrd=off  block_type=shift
  Shift3 : xbsIndex_r4/Shift  shift_dir=Right  shift_bits=CIC_shift_Tx  en=off  latency=0  precision=User Defined  arith_type="Signed  (2's comp)"  n_bits=17  bin_pt=14  quantization=Truncate  overflow=Wrap  dbl_ovrd=off  block_type=shift
  Terminator{,1..8} (9 alike) : Terminator
  Upsample CIC : xbsIndex_r4/Up Sample  sample_ratio=R_CIC  copy_samples=on  en=off  latency=0  dbl_ovrd=off  block_type=usamp
  Upsample CIC1 : xbsIndex_r4/Up Sample  sample_ratio=fCIC/(Rb/2)  copy_samples=on  en=off  latency=0  dbl_ovrd=off  block_type=usamp
  Upsample CIC2 : xbsIndex_r4/Up Sample  sample_ratio=R_CIC  copy_samples=on  en=off  latency=0  dbl_ovrd=off  block_type=usamp
  Upsample CIC3 : xbsIndex_r4/Up Sample  sample_ratio=R_CIC  copy_samples=on  en=off  latency=0  dbl_ovrd=off  block_type=usamp
  Upsample CIC4 : xbsIndex_r4/Up Sample  sample_ratio=fCIC/fHB  copy_samples=on  en=off  latency=0  dbl_ovrd=off  block_type=usamp
  Upsample CIC5 : xbsIndex_r4/Up Sample  sample_ratio=R_CIC  copy_samples=off  en=off  latency=0  dbl_ovrd=off  block_type=usamp
  Upsample CIC6 : xbsIndex_r4/Up Sample  sample_ratio=fCIC/fHB  copy_samples=on  en=off  latency=0  dbl_ovrd=off  block_type=usamp
  Upsample CICCOMP : xbsIndex_r4/Up Sample  sample_ratio=R_CICcomp  copy_samples=on  en=off  latency=0  dbl_ovrd=off  block_type=usamp
  Upsample CICCOMP1 : xbsIndex_r4/Up Sample  sample_ratio=R_CICcomp  copy_samples=on  en=off  latency=0  dbl_ovrd=off  block_type=usamp
  Upsample CICCOMP2 : xbsIndex_r4/Up Sample  sample_ratio=R_CICcomp  copy_samples=on  en=off  latency=0  dbl_ovrd=off  block_type=usamp
  Upsample CICCOMP3 : xbsIndex_r4/Up Sample  sample_ratio=R_CICcomp  copy_samples=off  en=off  latency=0  dbl_ovrd=off  block_type=usamp
  Upsample HB : xbsIndex_r4/Up Sample  sample_ratio=R_HB  copy_samples=on  en=off  latency=0  dbl_ovrd=off  block_type=usamp
  Upsample HB1 : xbsIndex_r4/Up Sample  sample_ratio=R_HB  copy_samples=on  en=off  latency=0  dbl_ovrd=off  block_type=usamp
  Upsample HB2 : xbsIndex_r4/Up Sample  sample_ratio=R_HB  copy_samples=on  en=off  latency=0  dbl_ovrd=off  block_type=usamp
  Upsample HB3 : xbsIndex_r4/Up Sample  sample_ratio=R_HB  copy_samples=off  en=off  latency=0  dbl_ovrd=off  block_type=usamp
  Upsample RRC : xbsIndex_r4/Up Sample  sample_ratio=R_RRC  copy_samples=on  en=off  latency=0  dbl_ovrd=off  block_type=usamp
  Upsample RRC1 : xbsIndex_r4/Up Sample  sample_ratio=R_RRC  copy_samples=on  en=off  latency=0  dbl_ovrd=off  block_type=usamp
  Upsample RRC2 : xbsIndex_r4/Up Sample  sample_ratio=R_RRC  copy_samples=on  en=off  latency=0  dbl_ovrd=off  block_type=usamp
  Upsample RRC3 : xbsIndex_r4/Up Sample  sample_ratio=R_RRC  copy_samples=off  en=off  latency=0  dbl_ovrd=off  block_type=usamp
  Interpolated : Outport
  tvalid_out : Outport  Port=2
  tlast_out : Outport  Port=3
  post_hb_data : Outport  Port=4
  post_hb_last : Outport  Port=5
  post_hb_valid : Outport  Port=6
  symbol_data : Outport  Port=7
  symbol_last : Outport  Port=8
  symbol_valid : Outport  Port=9
  wires:
  Mult/1 -> Mux1/2
  Mux1/1 -> post_hb_data/1
  Upsample CIC4/1 -> Mult1/1
  Mult1/1 -> Reinterpret/1
  Delay CIC3/1 -> Terminator6/1
  Delay HB1/1 -> Upsample CICCOMP/1, post_hb_valid/1
  Delay HB2/1 -> post_hb_last/1, Upsample CICCOMP3/1
  Constant/1 -> Mux/2
  Input_symbols/1 -> symbol_data/1, Convert1/1
  Mux/1 -> "FIR Compiler 7.2 "/1
  Delay CICCOMP2/1 -> Delay CIC4/1
  Delay CIC4/1 -> Upsample CIC5/1
  Delay CICCOMP1/1 -> Delay CIC2/1
  Delay CIC2/1 -> Upsample CIC/1
  Inverter/1 -> "CIC Compiler 4.0 "/2, FIR Compiler 7.2 2/2, "FIR Compiler 7.2 "/2, FIR Compiler 7.2 3/2
  Upsample CIC5/1 -> Delay CIC3/1
  Upsample RRC1/1 -> Upsample HB1/1, Delay RRC2/2, Delay RRC1/2
  Upsample RRC2/1 -> Upsample HB2/1, Delay RRC2/3, Delay RRC1/3
  Upsample HB1/1 -> Upsample CICCOMP1/1, Delay HB1/2, Delay HB2/2
  Upsample HB2/1 -> Upsample CICCOMP2/1, Delay HB1/3, Delay HB2/3
  Upsample CICCOMP1/1 -> Upsample CIC3/1, Delay CIC2/2, Delay CIC4/2, Delay CICCOMP1/2, Delay CICCOMP2/2
  Upsample CICCOMP2/1 -> Upsample CIC2/1, Delay CIC2/3, Delay CIC4/3, Delay CICCOMP1/3, Delay CICCOMP2/3
  tlast_in/1 -> symbol_last/1, Upsample RRC3/1
  Delay RRC1/1 -> Upsample HB3/1
  Upsample RRC3/1 -> Delay RRC1/1
  Upsample HB3/1 -> Delay HB2/1
  Upsample CICCOMP3/1 -> Delay CICCOMP2/1
  tready/1 -> Upsample RRC2/1
  Delay CIC1/1 -> Delay3/1, Logical1/1
  Upsample CICCOMP/1 -> Delay CICCOMP1/1
  Upsample HB/1 -> Delay HB1/1
  Upsample RRC/1 -> Delay RRC2/1
  Delay RRC2/1 -> Upsample HB/1
  tvalid_in/1 -> Mux/1, symbol_valid/1, Upsample RRC/1
  Upsample CIC3/1 -> Inverter/1, Delay4/2, Logical/1, Delay3/2, Delay5/2, Delay CIC1/2, Delay CIC3/2
  Upsample CIC2/1 -> "CIC Compiler 4.0 "/3, FIR Compiler 7.2 3/3, FIR Compiler 7.2 2/3, "FIR Compiler 7.2 "/3, Delay5/3, Delay3/3, Delay4/3, Logical1/2, Delay CIC1/3, Delay CIC3/3
  "CIC Compiler 4.0 "/2 -> Terminator8/1
  Upsample CIC/1 -> Delay CIC1/1
  Reset/1 -> Upsample RRC1/1
  Convert5/1 -> "CIC Compiler 4.0 "/1
  "CIC Compiler 4.0 "/1 -> Terminator7/1
  FIR Compiler 7.2 3/2 -> Terminator5/1
  FIR Compiler 7.2 3/1 -> Terminator4/1
  FIR Compiler 7.2 3/3 -> Convert5/1
  FIR Compiler 7.2 2/1 -> Terminator2/1
  FIR Compiler 7.2 2/2 -> Terminator3/1
  FIR Compiler 7.2 2/3 -> Shift/1
  "FIR Compiler 7.2 "/3 -> Convert4/1
  Shift3/1 -> CMult/1
  "FIR Compiler 7.2 "/2 -> Terminator1/1
  "FIR Compiler 7.2 "/1 -> Terminator/1
  PacketSize/1 -> Upsample CIC1/1
  Upsample CIC1/1 -> Relational/2
  Counter/1 -> Relational/1
  Logical/1 -> Counter/1
  Inverter1/1 -> Delay4/1, Logical/2
  Relational/1 -> Inverter1/1
  Delay4/1 -> tlast_out/1
  Delay3/1 -> tvalid_out/1
  Delay5/1 -> Interpolated/1
  Logical1/1 -> Counter/2
  "CIC Compiler 4.0 "/3 -> Shift3/1
  Convert4/1 -> FIR Compiler 7.2 2/1
  Convert1/1 -> Mux/3
  Shift/1 -> FIR Compiler 7.2 3/1, Mult/2, Mux1/3
  CMult/1 -> Mult1/2, Reinterpret1/1
  OutputGainStage/1 -> Upsample CIC4/1, Mult/1
  Reinterpret/1 -> Mux2/2
  Mux2/1 -> Delay5/1
  Reinterpret1/1 -> Mux2/3
  bypass_gain/1 -> Upsample CIC6/1, Mux1/1
  Upsample CIC6/1 -> Mux2/1

== system AXI_QPSK_Tx/AXI_QPSK_Generator/PostHB_Time_Domain/M_AXIS_SYMBOL_CTRL ==
  i_data : Inport
  tvalid_in : Inport  Port=2
  q_data : Inport  Port=3
  reset : Inport  Port=4
  packet_size : Inport  Port=5
  tready_in : Inport  Port=6
  transfer : Inport  Port=7
  auto_restart : Inport  Port=8
  AXI_Write_Interface : Subsystem
  Concat : xbsIndex_r4/Concat  num_inputs=2  dbl_ovrd=off  block_type=concat
  Reinterpret : xbsIndex_r4/Reinterpret  force_arith_type=on  arith_type=Unsigned  force_bin_pt=on  bin_pt=0  block_type=reinterpret
  Reinterpret1 : xbsIndex_r4/Reinterpret  force_arith_type=on  arith_type=Unsigned  force_bin_pt=on  bin_pt=0  block_type=reinterpret
  tdata_out : Outport
  tvalid_out : Outport  Port=2
  tlast_out : Outport  Port=3
  wires:
  AXI_Write_Interface/1(tdata_out) -> tdata_out/1
  AXI_Write_Interface/3(tvalid_out) -> tvalid_out/1
  AXI_Write_Interface/2(tlast_out) -> tlast_out/1
  tready_in/1 -> AXI_Write_Interface/7(tready)
  auto_restart/1 -> AXI_Write_Interface/3(auto_restart)
  transfer/1 -> AXI_Write_Interface/2(transfer)
  Concat/1 -> AXI_Write_Interface/5(tdata_in)
  reset/1 -> AXI_Write_Interface/1(int_reset)
  tvalid_in/1 -> AXI_Write_Interface/6(tvalid_in)
  packet_size/1 -> AXI_Write_Interface/4(packet_size)
  Reinterpret/1 -> Concat/1
  Reinterpret1/1 -> Concat/2
  q_data/1 -> Reinterpret/1
  i_data/1 -> Reinterpret1/1
